simulink model "Chapter_4_Section_3_Model"  (R2017a)
settings: Solver=ode4  StartTime=0.0  StopTime=200  FixedStep=stp_sz  MaxStep=.0001  MinStep=.00005  RelTol=1e-7  AbsTol=1e-7  EnableMultiTasking=on
InitFcn:
  | load Chapter_4_Section_3
  | warning off
StopFcn:
  | save data.mat u_simulation v_simulation psi_simulation r_simulation npr_user_provided npr_achievable alpha_user_provided alpha_achievable stp_sz
  | clear all
  | load('data.mat')
  | delete('data.mat')
values from neighbouring files (symbols this model uses):
  A_disk = 13.2025431267    [Chapter_4_Section_3.mat]
  a_r11 = [-0.000865667853776 -0.901318756108 0.00874486630837 -0.00765974060328 0.00955717632387 0.00641813989061 -0.011076069832 0.00201248118094 -0.00501952733262 0.00315605586996 -0.00210851076531 0.0148609220099 ... (324 elements, 18x18)]    [Chapter_4_Section_3.mat]
  a_r13 = [-0.0294995912119 -4.91037219533 -0.00332739568397 0.0888755061346 -0.00681796875441 0.183812407485 0.0112008036726 0.10429312155 -0.0251601482875 -0.228675692165 0.00453476042855 0.0594697753606 ... (169 elements, 13x13)]    [Chapter_4_Section_3.mat]
  a_r15 = [-0.00127786555898 0.776225741104 -0.00474776997752 -0.00131066749835 0.0137520402687 -0.00211384579247 8.8019955143e-05 -0.00028996241197 -0.00129826872567 -0.0202543144732 0.0030370404199 -0.00453425604591 ... (169 elements, 13x13)]    [Chapter_4_Section_3.mat]
  a_r22 = [-0.000797108949019 -1.01015556887 0.00406573750109 -0.00111578544774 0.00423859757219 -0.00799128279013 0.00569024815652 -0.0167562674532 0.00334935655618 -0.000712432292804 0.00154242142086 0.00240437743229 ... (169 elements, 13x13)]    [Chapter_4_Section_3.mat]
  a_r24 = [-0.000686927823555 -0.95665602689 0.00244839898375 0.00145613314595 -0.00607023426216 0.0163996841317 0.00152022458075 -0.000736874734971 -0.00294919321651 -0.000761800577268 -0.00251686123035 -0.00197732815976 ... (169 elements, 13x13)]    [Chapter_4_Section_3.mat]
  a_r26 = [-0.194397873228 1.89810259721 -0.0873186628061 -0.241231729519 0.281206161775 -0.16994038615 -0.116565511469 -0.0496572593209 0.0216084469732 0.0912933167406 0.0299797727001 0.0314987707028 ... (169 elements, 13x13)]    [Chapter_4_Section_3.mat]
  a_r31 = [-0.00489112559449 -3.89960530455 -0.0361162658575 0.0265931197764 0.0034376033088 0.000316401308368 -0.0243996243526 0.0792200139858 -0.023187698537 -0.0726743997029 0.00400632061963 -0.0350516560041 ... (169 elements, 13x13)]    [Chapter_4_Section_3.mat]
  a_r33 = [-0.601431448276 0.50360246711 0.500115950342 -0.0452293844892 -0.0181314142185 -0.0323524621531 0.0355826051968 0.0329239610677 0.0940919952313 0.0566642992805 -0.0379178935102 0.0254835488846 ... (169 elements, 13x13)]    [Chapter_4_Section_3.mat]
  a_r35 = [-0.861988746714 -0.582511154549 0.34264856173 -0.0655310417272 -0.417167685168 0.183176698588 -0.473887691644 -0.225677727522 -0.133571139717 -0.218168843707 0.0850592077583 -0.0257492082836 ... (169 elements, 13x13)]    [Chapter_4_Section_3.mat]
  a_r42 = [-0.000411079312172 -0.966350953459 0.00419936729713 0.00358740198521 -0.00356571428733 -0.00958951498266 -0.00230062261745 -3.48708248632e-05 -0.00350313209064 -0.00772126326768 -0.0011918234528 -0.00149424537901 ... (169 elements, 13x13)]    [Chapter_4_Section_3.mat]
  a_r44 = [-0.000156115728087 -0.944139704333 -0.00242185567679 0.00620214191605 0.00232565005277 -0.00625050722164 0.00126021167241 -0.000681873506535 0.0011931592381 -0.00289361611357 -0.00138182415247 -0.00252837386868 ... (169 elements, 13x13)]    [Chapter_4_Section_3.mat]
  a_r46 = [-0.000218462457517 1.89677852742 0.00896242354968 -0.00290259500747 0.00225128874867 0.00254539590487 0.00120681433209 0.00261900930035 0.00149629742842 0.000796832004109 0.00199591847947 0.00352664402036 ... (169 elements, 13x13)]    [Chapter_4_Section_3.mat]
  a_r51 = [-0.0010898880101 0.776080724329 0.000225388678941 0.00375234840616 -0.00838297691459 -0.00447310416982 -0.0119510882322 -0.00692765468718 0.00227273345413 -0.0063592610709 0.000914007544175 0.00943534814934 ... (169 elements, 13x13)]    [Chapter_4_Section_3.mat]
  a_r53 = [-0.83377539904 0.569677058563 0.434285019976 0.157205409215 -0.397195569542 -0.255164078245 -0.141246880777 0.177451291189 -0.182828550566 0.0648162508754 0.244251292681 0.160100487197 ... (169 elements, 13x13)]    [Chapter_4_Section_3.mat]
  a_r55 = [-0.000352406331634 0.764343029796 0.00339830320259 -0.000678251137483 -0.00243783779313 -0.00215979913278 0.00196909451093 -0.00577428819561 -0.00349811892924 -0.00488920883323 0.00112064970343 0.000774855197444 ... (169 elements, 13x13)]    [Chapter_4_Section_3.mat]
  a_r62 = [-0.546519039316 -1.22303009993 0.393735845548 -0.120016588191 0.38151861373 -0.213578592342 -0.602267954372 -0.105716444149 -0.153151371839 -0.163939447448 -0.555540353196 0.0685401630267 ... (169 elements, 13x13)]    [Chapter_4_Section_3.mat]
  a_r64 = [-0.0406191100017 -5.18251105957 -0.115497941507 -0.0935821370219 0.180972853448 -0.0201998949456 -0.0698170640352 -0.0736823539521 -0.034828919888 0.0876659960431 -0.0419335596239 -0.0240984963396 ... (169 elements, 13x13)]    [Chapter_4_Section_3.mat]
  a_r66 = [-0.00276803466684 1.11530008029 0.0229779449181 0.0262185319857 0.00628472844795 0.000156167369042 -0.00250093023805 -0.0114435042874 -0.00826774415326 -0.00991601759993 -0.00812142854996 0.0148245002111 ... (169 elements, 13x13)]    [Chapter_4_Section_3.mat]
  A_rudder = 6    [Chapter_4_Section_3.mat]
  alpha_max = 0.392699081699    [Chapter_4_Section_3.mat]
  b_r11 = [-1.91804272115 -67.7547902158 12.3212653748 -6.25011871643 13.082442224 5.48501776184 -10.1596546398 2.56004852009 -4.74360113798 3.95981895348 -2.02856412397 18.3264246889 ... (18 elements, 18x1)]    [Chapter_4_Section_3.mat]
  b_r13 = [9.68113335046 8.54720242819 0.883931047444 -5.56576078332 1.72641800243 -13.8756826027 -2.702777864 -9.4621991361 5.92943514782 22.6516835054 -1.0074598861 -6.31102592982 ... (13 elements, 13x1)]    [Chapter_4_Section_3.mat]
  b_r22 = [-8.230214728 -263.156134326 24.2327808151 -4.87921448873 19.1715641288 -45.8768653263 26.6325387064 -91.9399975548 16.6663243552 -3.80929112747 7.68030110892 12.8381492859 ... (13 elements, 13x1)]    [Chapter_4_Section_3.mat]
  b_r24 = [20.6689502907 674.321335078 -41.3637763247 -19.2444203625 82.0775505272 -259.897803047 -22.2545830602 11.3827604156 43.2189922355 11.7516897475 36.9394390446 30.4503929007 ... (13 elements, 13x1)]    [Chapter_4_Section_3.mat]
  b_r26 = [206.794755218 -62.242559329 24.5666904254 184.158146246 -103.419961827 115.160111337 76.4499795128 20.3457431208 -13.1704465249 -41.5730935141 -18.1334448714 -14.4641153742 ... (13 elements, 13x1)]    [Chapter_4_Section_3.mat]
  b_r31 = [3.76230189948 5.16928151238 2.64945725635 -18.4251953385 -2.0625905672 -0.18887543415 4.20433084471 -14.07893046 13.0563354882 16.4007691754 -2.13849071942 8.28528512456 ... (13 elements, 13x1)]    [Chapter_4_Section_3.mat]
  b_r33 = [-425.265727934 16.4952177922 163.76327445 -15.539902078 -6.59006558263 -11.1862310226 12.8543123126 11.4260264426 33.8206936715 19.7626944669 -13.5783728882 8.91023495161 ... (13 elements, 13x1)]    [Chapter_4_Section_3.mat]
  b_r35 = [955.467057384 23.8174564739 -126.402446683 48.3788727465 168.435579445 -128.161344325 216.24493699 142.979450788 65.1193355403 134.911935543 -50.7648858119 13.1799100865 ... (13 elements, 13x1)]    [Chapter_4_Section_3.mat]
  b_r42 = [15.9360311823 665.959154186 -98.5777560157 -55.5400651809 61.9220987195 200.312325561 47.5124103398 0.631683490985 64.1219861023 155.750535985 22.3985447876 29.803792586 ... (13 elements, 13x1)]    [Chapter_4_Section_3.mat]
  b_r44 = [-27.1891200017 -1761.50772747 -283.391471232 367.311489951 182.522124626 -579.755911925 104.353356772 -62.2376848714 99.3185259533 -260.784153955 -116.536414334 -226.454300618 ... (13 elements, 13x1)]    [Chapter_4_Section_3.mat]
  b_r46 = [-26.6906838426 431.487773123 657.709356633 -144.976364483 114.646575538 180.775978583 85.0953284375 135.592940904 78.9082960716 55.2973047721 106.740201988 241.432567993 ... (13 elements, 13x1)]    [Chapter_4_Section_3.mat]
  b_r51 = [-27.9768378982 741.05041888 2.33758926296 57.3995096963 -127.005620965 -47.2947833409 -133.876425682 -98.5907202753 26.0445243962 -88.3721242204 10.7680008324 130.122749963 ... (13 elements, 13x1)]    [Chapter_4_Section_3.mat]
  b_r53 = [949.455593416 -23.2452293814 -157.318364745 -121.412853107 173.067821874 177.10214052 64.7164189373 -120.452255472 86.0623964314 -43.0643550932 -116.39314584 -105.497696438 ... (13 elements, 13x1)]    [Chapter_4_Section_3.mat]
  b_r55 = [-217.127382907 9506.32343029 1148.82922273 -188.742556573 -694.43970838 -709.996440288 566.872400877 -1877.38940059 -1026.37679575 -1566.80129668 332.089563592 247.692614281 ... (13 elements, 13x1)]    [Chapter_4_Section_3.mat]
  b_r62 = [259.61149635 16.5485296799 -38.0095496792 45.1883806678 -40.3107166739 78.3455844965 73.5107367495 37.0054960802 51.6709447748 22.7410486275 84.4875008959 -21.9559289205 ... (13 elements, 13x1)]    [Chapter_4_Section_3.mat]
  b_r64 = [156.539833252 187.686482031 376.820920142 59.4312894666 -548.902692032 17.0176436095 70.7484878223 206.821047291 37.1716677759 -243.032149857 114.824775027 27.0037475025 ... (13 elements, 13x1)]    [Chapter_4_Section_3.mat]
  b_r66 = [-314.266256408 5285.46587095 1093.01941502 1627.30071258 387.633965073 8.0986510694 -130.443621448 -701.343286032 -436.49966457 -600.0481003 -433.735518303 884.367320612 ... (13 elements, 13x1)]    [Chapter_4_Section_3.mat]
  bettas_CQ = [0 5.39 17.77 34.97 50.79 58.7 64.55 68.33 73.49 85.2 93.11 102.75 ... (40 elements, 1x40)]    [Chapter_4_Section_3.mat]    (also in looking_up_n.m = [0 5.39 17.77 34.97 50.79 58.7 64.55 68.33 73.49 85.2 93.11 )
  bettas_CT = [0 5.37 16.73 33.6 44.63 60.82 73.22 80.46 86.3 92.15 100.41 110.74 ... (52 elements, 1x52)]    [Chapter_4_Section_3.mat]    (also in looking_up_n.m = [0 5.37 16.73 33.6 44.63 60.82 73.22 80.46 86.3 92.15 100.41)
  c_r11 = [1.91804272142 -67.7547902158 -12.3212653748 -6.25011871643 -13.082442224 5.48501776185 -10.1596546398 -2.56004852009 -4.74360113798 -3.95981895348 -2.02856412396 -18.3264246889 ... (18 elements, 1x18)]    [Chapter_4_Section_3.mat]
  c_r13 = [9.68113335045 -8.54720242824 0.883931047418 5.56576078332 1.72641800244 13.8756826027 -2.702777864 9.4621991361 5.92943514781 -22.6516835054 -1.0074598861 6.31102592982 ... (13 elements, 1x13)]    [Chapter_4_Section_3.mat]
  c_r22 = [8.23021472807 -263.156134326 -24.2327808151 -4.87921448871 19.1715641288 45.8768653263 26.6325387064 91.9399975548 16.6663243552 3.80929112749 7.68030110892 -12.8381492859 ... (13 elements, 1x13)]    [Chapter_4_Section_3.mat]
  c_r24 = [20.6689502903 -674.321335078 -41.3637763247 19.2444203625 -82.0775505271 -259.897803047 22.2545830602 11.3827604156 -43.2189922355 11.7516897475 -36.9394390446 30.4503929007 ... (13 elements, 1x13)]    [Chapter_4_Section_3.mat]
  c_r26 = [-206.794755218 -62.2425593289 24.5666904254 -184.158146246 -103.419961827 -115.160111337 -76.4499795128 20.3457431209 13.1704465249 -41.5730935141 18.1334448714 -14.4641153742 ... (13 elements, 1x13)]    [Chapter_4_Section_3.mat]
  c_r31 = [3.76230189951 -5.16928151238 -2.64945725636 -18.4251953385 -2.0625905672 -0.188875434257 -4.2043308447 14.07893046 13.0563354882 -16.4007691754 -2.13849071943 -8.28528512456 ... (13 elements, 1x13)]    [Chapter_4_Section_3.mat]
  c_r33 = [-425.265727934 -16.4952177923 -163.76327445 15.539902078 -6.5900655826 11.1862310226 12.8543123126 -11.4260264426 33.8206936715 -19.7626944669 -13.5783728882 -8.91023495161 ... (13 elements, 1x13)]    [Chapter_4_Section_3.mat]
  c_r35 = [-955.467057384 23.8174564746 -126.402446683 -48.3788727464 168.435579445 128.161344325 216.24493699 -142.979450788 65.1193355403 -134.911935543 50.7648858119 13.1799100865 ... (13 elements, 1x13)]    [Chapter_4_Section_3.mat]
  c_r42 = [15.9360311824 -665.959154186 -98.5777560157 55.5400651809 -61.9220987195 200.312325561 47.5124103398 -0.631683490192 -64.1219861023 155.750535985 -22.3985447876 29.803792586 ... (13 elements, 1x13)]    [Chapter_4_Section_3.mat]
  c_r44 = [27.189120009 -1761.50772747 283.391471232 367.311489951 182.522124626 579.755911925 104.353356772 62.2376848713 99.3185259533 260.784153955 -116.536414334 226.454300618 ... (13 elements, 1x13)]    [Chapter_4_Section_3.mat]
  c_r46 = [26.6906838375 431.487773123 -657.709356633 -144.976364484 114.646575538 -180.775978583 -85.0953284373 135.592940904 78.9082960717 -55.297304772 106.740201988 -241.432567993 ... (13 elements, 1x13)]    [Chapter_4_Section_3.mat]
  c_r51 = [27.9768378982 741.05041888 2.33758926325 -57.3995096963 127.005620965 -47.2947833409 -133.876425682 98.5907202753 26.0445243962 88.3721242204 10.7680008324 -130.122749963 ... (13 elements, 1x13)]    [Chapter_4_Section_3.mat]
  c_r53 = [-949.455593416 -23.2452293814 -157.318364745 121.412853107 173.067821874 -177.10214052 64.7164189374 120.452255472 86.0623964314 43.0643550932 -116.39314584 105.497696438 ... (13 elements, 1x13)]    [Chapter_4_Section_3.mat]
  c_r55 = [217.12738291 9506.32343029 -1148.82922273 -188.742556576 -694.43970838 709.996440288 566.872400876 1877.38940059 -1026.37679575 1566.80129668 332.089563594 -247.69261428 ... (13 elements, 1x13)]    [Chapter_4_Section_3.mat]
  c_r62 = [-259.61149635 16.5485296799 -38.0095496792 -45.1883806678 -40.3107166739 -78.3455844965 73.5107367495 -37.0054960802 -51.6709447748 22.7410486275 84.4875008959 21.9559289205 ... (13 elements, 1x13)]    [Chapter_4_Section_3.mat]
  c_r64 = [-156.539833251 187.686482031 -376.820920142 59.4312894666 548.902692032 17.0176436097 70.7484878223 -206.82104729 37.1716677758 243.032149857 -114.824775027 27.0037475025 ... (13 elements, 1x13)]    [Chapter_4_Section_3.mat]
  c_r66 = [314.266256408 5285.46587095 1093.01941502 -1627.30071258 -387.633965073 8.09865107118 -130.443621448 701.343286032 -436.49966457 600.0481003 -433.735518303 -884.367320612 ... (13 elements, 1x13)]    [Chapter_4_Section_3.mat]
  CQs = [0.008 0.007 -0.002 -0.018 -0.037 -0.049 -0.06 -0.065 -0.068 -0.059 -0.057 -0.059 ... (40 elements, 1x40)]    [Chapter_4_Section_3.mat]    (also in looking_up_n.m = -0.1.*[-0.08 -0.07 0.02 0.18 0.37 0.49 0.6 0.65 0.68 0.59 0.)
  CTs = [0.32 0.29 0.19 0.01 -0.16 -0.46 -0.7 -0.77 -0.7 -0.63 -0.63 -0.69 ... (52 elements, 1x52)]    [Chapter_4_Section_3.mat]    (also in looking_up_n.m = [0.32 0.29 0.19 0.01 -0.16 -0.46 -0.7 -0.77 -0.7 -0.63 -0.63)
  d_r11 = 95.5285227708    [Chapter_4_Section_3.mat]
  d_r13 = -14.1628545989    [Chapter_4_Section_3.mat]
  d_r22 = 1468.51041279    [Chapter_4_Section_3.mat]
  d_r24 = -9785.77027698    [Chapter_4_Section_3.mat]
  d_r26 = -1700.92421833    [Chapter_4_Section_3.mat]
  d_r31 = -0.95522945761    [Chapter_4_Section_3.mat]
  d_r33 = 3827.81220596    [Chapter_4_Section_3.mat]
  d_r35 = -19539.5268707    [Chapter_4_Section_3.mat]
  d_r42 = -9418.04264727    [Chapter_4_Section_3.mat]
  d_r44 = 68252.1479072    [Chapter_4_Section_3.mat]
  d_r46 = -10162.1377852    [Chapter_4_Section_3.mat]
  d_r51 = 12054.4514237    [Chapter_4_Section_3.mat]
  d_r53 = -19539.5038011    [Chapter_4_Section_3.mat]
  d_r55 = 1991036.95813    [Chapter_4_Section_3.mat]
  d_r62 = -1405.47636444    [Chapter_4_Section_3.mat]
  d_r64 = -12342.2523681    [Chapter_4_Section_3.mat]
  d_r66 = 610786.440495    [Chapter_4_Section_3.mat]
  DEN = 5.34671106464e+28    [Chapter_4_Section_3.mat]
  dist_LOS = [-50 -49 -48 -47 -46 -45 -44 -43 -42 -41 -40 -39 ... (1051 elements, 1x1051)]    [Chapter_4_Section_3.mat]
  Dpr = 4.1    [Chapter_4_Section_3.mat]    (also in looking_up_n.m = u(4))
  Dw = 0.110526315789    [Chapter_4_Section_3.mat]
  dx = 10    [Chapter_4_Section_3.mat]
  dxr = 48.75    [Chapter_4_Section_3.mat]
  dy = 2    [Chapter_4_Section_3.mat]
  dz = 0.8    [Chapter_4_Section_3.mat]
  dzr = 0.514285714286    [Chapter_4_Section_3.mat]
  g = 10    [Chapter_4_Section_3.mat]
  gravity = 10    [Chapter_4_Section_3.mat]
  INDEX = [1 2 3 4 5 6 7 8 9]    [Chapter_4_Section_3.mat]
  Ix = 724554000    [Chapter_4_Section_3.mat]
  Iy = 4528460000    [Chapter_4_Section_3.mat]
  Iz = 4528460000    [Chapter_4_Section_3.mat]
  k_wave = [0.0157865285852 0.0224311321394 0.0345394916241 0.0578593033576 0.0778685019714 0.0983501894009 0.10403521245 0.134043066308 0.155236404606 0.203205074918 0.220032771713 0.262178651673 ... (20 elements, 1x20)]    [Chapter_4_Section_3.mat]
  Last_Pt_Accuracy = 30    [Chapter_4_Section_3.mat]
  LBP = 100    [Chapter_4_Section_3.mat]
  m = 7264000    [Chapter_4_Section_3.mat]
  phase = [4.61787442739 6.09845039199 5.44708367148 0.54182753101 2.30238916367 2.31974450279 4.30416083443 3.75697809799 4.95971993271 2.31003141527 1.29451121971 0.54454197722 ... (20 elements, 1x20)]    [Chapter_4_Section_3.mat]
  phi_0 = 0    [Chapter_4_Section_3.mat]
  psi_0 = 0    [Chapter_4_Section_3.mat]
  R_convrg = 220    [Chapter_4_Section_3.mat]
  radius_LOS = [166.575605377 166.637026665 166.698699321 166.760625342 166.82280675 166.885245588 166.947943925 167.010903854 167.074127493 167.137616985 167.201374499 167.265402228 ... (1051 elements, 1x1051)]    [Chapter_4_Section_3.mat]
  raw = 1000    [Chapter_4_Section_3.mat]    (also in looking_up_n.m = u(3))
  s = 0.15    [Chapter_4_Section_3.mat]
  S11 = 5.22457985714e+28    [Chapter_4_Section_3.mat]
  S13 = 3.79917831589e+26    [Chapter_4_Section_3.mat]
  S15 = -4.97006200608e+19    [Chapter_4_Section_3.mat]
  S22 = 4.58630932583e+28    [Chapter_4_Section_3.mat]
  S24 = 9.38800137353e+19    [Chapter_4_Section_3.mat]
  S26 = 1.30387886946e+18    [Chapter_4_Section_3.mat]
  S31 = 3.83422033136e+26    [Chapter_4_Section_3.mat]
  S33 = 1.77296018417e+28    [Chapter_4_Section_3.mat]
  S35 = 2.44593333777e+19    [Chapter_4_Section_3.mat]
  S42 = 8.93369784557e+19    [Chapter_4_Section_3.mat]
  S44 = 7.37931315974e+19    [Chapter_4_Section_3.mat]
  S46 = 27990784014.6    [Chapter_4_Section_3.mat]
  S51 = -4.98658939538e+19    [Chapter_4_Section_3.mat]
  S53 = 2.45188465874e+19    [Chapter_4_Section_3.mat]
  S55 = 1.18069051188e+19    [Chapter_4_Section_3.mat]
  S62 = 1.30580221388e+18    [Chapter_4_Section_3.mat]
  S64 = 23535167243.9    [Chapter_4_Section_3.mat]
  S66 = 1.18069078235e+19    [Chapter_4_Section_3.mat]
  ... (+18 more)
undefined symbols (not defined in the file or in its folder): magnitude
libraries: simulink x9
(part 6 of 6)

== system Chapter_4_Section_3_Model/Ship_Model/Ship Dynamics with Environmental Forces and Memory Effect/Buoyancy_Forces/Subsystem/wave elevation from multiple frequencies/Seakeeping motion of the ship from RAO's and wave spectrum /Sea wave elevation from  ==
  w_star : Inport
  k_wave : Inport  Port=2
  phase : Inport  Port=3
  X : Inport  Port=4
  Y : Inport  Port=5
  t : Inport  Port=6
  S_power of ith wave : Inport  Port=7
  ksi : Inport  Port=8
  Math Function : Math  Operator=sqrt  SaturateOnIntegerOverflow=on
  Product{,2..5} (5 alike) : Product  RndMeth=Zero
  Product1 : Product  Inputs=3  RndMeth=Zero
  Read Me : simulink/Model-Wide Utilities/DocBlock  DocumentType=Text
  Sum : Sum  Inputs=|+|+|-|
  Sum1 : Sum  Inputs=|+|+|
  Trigonometric Function : Trigonometry  Operator=cos
  Trigonometric Function1 : Trigonometry
  Trigonometric Function2 : Trigonometry  Operator=cos
  transforming Y to the z-upward -inertial frame(our inertial frame has z-downwards) : Gain  Gain=-1
  transforming the wave elevation from wave frame to  our inertial frame that has z-downwards : Gain  Gain=-1
  w12 : Constant  Value=2
  w13 : Constant  Value=Dw
  Sea wave Elevation(m) : Outport
  wires:
  transforming the wave elevation from wave frame to  our inertial frame that has z-downwards/1 -> Sea wave Elevation(m)/1
  transforming Y to the z-upward -inertial frame(our inertial frame has z-downwards)/1 -> [Y]
  Product5/1 -> transforming the wave elevation from wave frame to  our inertial frame that has z-downwards/1
  Trigonometric Function2/1 -> Product5/2
  Math Function/1 -> Product5/1
  Product1/1 -> Math Function/1
  [Dw] -> Product1/3
  [S] -> Product1/2
  w12/1 -> Product1/1
  Sum/1 -> Trigonometric Function2/1
  w13/1 -> [Dw]
  Product4/1 -> Sum/3
  [k_wave] -> Product4/1
  Sum1/1 -> Product4/2
  Product3/1 -> Sum1/2
  Product2/1 -> Sum1/1
  Trigonometric Function1/1 -> Product3/2
  [Y] -> Product3/1
  Trigonometric Function/1 -> Product2/2
  [X] -> Product2/1
  ksi/1 -> Trigonometric Function/1, Trigonometric Function1/1
  Y/1 -> transforming Y to the z-upward -inertial frame(our inertial frame has z-downwards)/1
  X/1 -> [X]
  phase/1 -> [phase]
  k_wave/1 -> [k_wave]
  w_star/1 -> [w_star]
  [phase] -> Sum/2
  Product/1 -> Sum/1
  [t] -> Product/2
  [w_star] -> Product/1
  t/1 -> [t]
  S_power of ith wave/1 -> [S]

== system Chapter_4_Section_3_Model/Ship_Model/Ship Dynamics with Environmental Forces and Memory Effect/Buoyancy_Forces/Subsystem/wave elevation from multiple frequencies1/Seakeeping motion of the ship from RAO's and wave spectrum /Sea wave elevation from  ==
  w_star : Inport
  k_wave : Inport  Port=2
  phase : Inport  Port=3
  X : Inport  Port=4
  Y : Inport  Port=5
  t : Inport  Port=6
  S_power of ith wave : Inport  Port=7
  ksi : Inport  Port=8
  Math Function : Math  Operator=sqrt  SaturateOnIntegerOverflow=on
  Product{,2..5} (5 alike) : Product  RndMeth=Zero
  Product1 : Product  Inputs=3  RndMeth=Zero
  Read Me : simulink/Model-Wide Utilities/DocBlock  DocumentType=Text
  Sum : Sum  Inputs=|+|+|-|
  Sum1 : Sum  Inputs=|+|+|
  Trigonometric Function : Trigonometry  Operator=cos
  Trigonometric Function1 : Trigonometry
  Trigonometric Function2 : Trigonometry  Operator=cos
  transforming Y to the z-upward -inertial frame(our inertial frame has z-downwards) : Gain  Gain=-1
  transforming the wave elevation from wave frame to  our inertial frame that has z-downwards : Gain  Gain=-1
  w12 : Constant  Value=2
  w13 : Constant  Value=Dw
  Sea wave Elevation(m) : Outport
  wires:
  transforming the wave elevation from wave frame to  our inertial frame that has z-downwards/1 -> Sea wave Elevation(m)/1
  transforming Y to the z-upward -inertial frame(our inertial frame has z-downwards)/1 -> [Y]
  Product5/1 -> transforming the wave elevation from wave frame to  our inertial frame that has z-downwards/1
  Trigonometric Function2/1 -> Product5/2
  Math Function/1 -> Product5/1
  Product1/1 -> Math Function/1
  [Dw] -> Product1/3
  [S] -> Product1/2
  w12/1 -> Product1/1
  Sum/1 -> Trigonometric Function2/1
  w13/1 -> [Dw]
  Product4/1 -> Sum/3
  [k_wave] -> Product4/1
  Sum1/1 -> Product4/2
  Product3/1 -> Sum1/2
  Product2/1 -> Sum1/1
  Trigonometric Function1/1 -> Product3/2
  [Y] -> Product3/1
  Trigonometric Function/1 -> Product2/2
  [X] -> Product2/1
  ksi/1 -> Trigonometric Function/1, Trigonometric Function1/1
  Y/1 -> transforming Y to the z-upward -inertial frame(our inertial frame has z-downwards)/1
  X/1 -> [X]
  phase/1 -> [phase]
  k_wave/1 -> [k_wave]
  w_star/1 -> [w_star]
  [phase] -> Sum/2
  Product/1 -> Sum/1
  [t] -> Product/2
  [w_star] -> Product/1
  t/1 -> [t]
  S_power of ith wave/1 -> [S]

== matlab function Chapter_4_Section_3_Model/Ship_Model/Ship Dynamics with Environmental Forces and Memory Effect/Six DOF State Integrator of the Ship/J2 matrix ==
  data: u input; y output
function y = J2(u)
% This block supports an embeddable subset of the MATLAB language.
% See the help menu for details. 
y=[1 sin(u(1))*tan(u(2)) cos(u(1))*tan(u(2));0 cos(u(1)) -sin(u(1));0 sin(u(1))/cos(u(2)) cos(u(1))/cos(u(2))];

== matlab function Chapter_4_Section_3_Model/Ship_Model/Ship Dynamics with Environmental Forces and Memory Effect/Six DOF State Integrator of the Ship/J1 matrix ==
  data: u input; y output
function y = J1(u)
% This block supports an embeddable subset of the MATLAB language.
% See the help menu for details. 
y=[cos(u(3))*cos(u(2))    -sin(u(3))*cos(u(1))+cos(u(3))*sin(u(2))*sin(u(1))   sin(u(3))*sin(u(1))+cos(u(3))*cos(u(1))*sin(u(2))  ;    ...
    sin(u(3))*cos(u(2))           cos(u(3))*cos(u(1))+ sin(u(1))*sin(u(2))*sin(u(3))    -cos(u(3))*sin(u(1))+sin(u(2))*sin(u(3))*cos(u(1))  ; ... 
-sin(u(2))                                             cos(u(2))*sin(u(1))                                                                 cos(u(2))*cos(u(1)) ];

== matlab function Chapter_4_Section_3_Model/Ship_Model/Ship Dynamics with Environmental Forces and Memory Effect/Buoyancy_Forces/J1 matrix ==
  data: u input; y output
function y = J1(u)
% This block supports an embeddable subset of the MATLAB language.
% See the help menu for details. 
y=inv(u);

== matlab function Chapter_4_Section_3_Model/Ship_Model/Ship Dynamics with Environmental Forces and Memory Effect/Wave Excitation Force/wave elevation from multiple frequencies2/Seakeeping motion of the ship from RAO's and wave spectrum /Embedded MATLAB Function ==
  data: index input; y output; A input
function y = fcn(index,A)
% This block supports an embeddable subset of the MATLAB language.
% See the help menu for details. 
y =A(index);

== matlab function Chapter_4_Section_3_Model/Ship_Model/Ship Dynamics with Environmental Forces and Memory Effect/Wave Excitation Force/wave elevation from multiple frequencies2/Seakeeping motion of the ship from RAO's and wave spectrum /Embedded MATLAB Function1 ==
  data: index input; y output; A input
function y = fcn(index,A)
% This block supports an embeddable subset of the MATLAB language.
% See the help menu for details. 
y =A(index);

== matlab function Chapter_4_Section_3_Model/Ship_Model/Ship Dynamics with Environmental Forces and Memory Effect/Buoyancy_Forces/Subsystem/wave elevation from multiple frequencies1/Seakeeping motion of the ship from RAO's and wave spectrum /Embedded MATLAB Function ==
  data: index input; y output; A input
function y = fcn(index,A)
% This block supports an embeddable subset of the MATLAB language.
% See the help menu for details. 
y =A(index);

== matlab function Chapter_4_Section_3_Model/Ship_Model/Ship Dynamics with Environmental Forces and Memory Effect/Buoyancy_Forces/Subsystem/wave elevation from multiple frequencies1/Seakeeping motion of the ship from RAO's and wave spectrum /Embedded MATLAB Function1 ==
  data: index input; y output; A input
function y = fcn(index,A)
% This block supports an embeddable subset of the MATLAB language.
% See the help menu for details. 
y =A(index);

== matlab function Chapter_4_Section_3_Model/Ship_Model/Ship Dynamics with Environmental Forces and Memory Effect/Buoyancy_Forces/Subsystem/J1 matrix ==
  data: u input; y output
function y = J1(u)
% This block supports an embeddable subset of the MATLAB language.
% See the help menu for details. 
y=u(1,:)   ;

== matlab function Chapter_4_Section_3_Model/Ship_Model/Ship Dynamics with Environmental Forces and Memory Effect/Buoyancy_Forces/Subsystem/J1 matrix1 ==
  data: u input; y output
function y = J1(u)
% This block supports an embeddable subset of the MATLAB language.
% See the help menu for details. 
y=u(2,:)   ;

== matlab function Chapter_4_Section_3_Model/Ship_Model/Ship Dynamics with Environmental Forces and Memory Effect/Buoyancy_Forces/Subsystem/wave elevation from multiple frequencies1/Seakeeping motion of the ship from RAO's and wave spectrum /Embedded MATLAB Function2 ==
  data: index input; y output; A input
function y = fcn(index,A)
% This block supports an embeddable subset of the MATLAB language.
% See the help menu for details. 
y =A(index);

== matlab function Chapter_4_Section_3_Model/Ship_Model/Ship Dynamics with Environmental Forces and Memory Effect/Wave Excitation Force/wave elevation from multiple frequencies2/Seakeeping motion of the ship from RAO's and wave spectrum /Embedded MATLAB Function2 ==
  data: index input; y output; A input
function y = fcn(index,A)
% This block supports an embeddable subset of the MATLAB language.
% See the help menu for details. 
y =A(index);

== matlab function Chapter_4_Section_3_Model/Ship_Model/LOS2/Breivik Model for psi/pi2inf ==
  data: x_los input; state_k output; y_los input; x input; y input; state_k_1 input; psi_k_1 input; psi_k input; accumulation_k_1 input; accumulation_k output
function [state_k ,accumulation_k]= fcn(x_los,y_los,x,y,state_k_1,psi_k_1,psi_k,accumulation_k_1)
delta_x = x_los - x;
delta_y = y_los- y;


% initialize:
accumulation_k = accumulation_k_1;
state_k=state_k_1;
% if( sign(delta_y)==1 && sign(delta_x)==1 )
if( sign(delta_y)>=0 && sign(delta_x)>=0 )
    % Now in the 1.quadrant
    state_k=1;
    if(state_k_1==3)
        if( (psi_k+abs(psi_k_1))<=pi )
            accumulate = psi_k - psi_k_1;
        else
            accumulate = psi_k_1 - psi_k + 2*pi;
        end
    else % state_k_1 == 1, 2 or 4
        accumulate = psi_k - psi_k_1;
    end
% elseif ( sign(delta_y)==-1 && sign(delta_x)==1 )
elseif ( sign(delta_y)<=0 && sign(delta_x)>=0 )
    % Now in the 2.quadrant
    state_k=2;
    if(state_k_1==4)
        if( (abs(psi_k)+psi_k_1)<=pi )
            accumulate = psi_k - psi_k_1;
        else
            accumulate = psi_k - psi_k_1 + 2*pi;
        end
    else % state_k_1 == 1, 2 or 3
        accumulate = psi_k - psi_k_1;
    end
% elseif (sign(delta_y)==-1 && sign(delta_x)==-1 )
elseif (sign(delta_y)<0 && sign(delta_x)<=0 )
    % Now in the 3.quadrant
    state_k=3;
    if(state_k_1==1)
        if( (abs(psi_k)+psi_k_1)<=pi )
            accumulate = psi_k - psi_k_1;
        else
            accumulate = psi_k - psi_k_1 + 2*pi;
        end
    elseif(state_k_1==4)
        accumulate = psi_k - psi_k_1 + 2*pi;
    else % state_k_1 == 2 or 3
        accumulate = psi_k - psi_k_1;
    end
else
    % sign(delta_y)==1 && sign(delta_x)==-1
    % Now in the 4.quadrant
    state_k=4;
    if(state_k_1==2)
        if( (psi_k+abs(psi_k_1))<=pi )
            accumulate = psi_k - psi_k_1;
        else
            accumulate = psi_k_1 - psi_k + 2*pi;
        end
    elseif(state_k_1==3)
        accumulate = psi_k - psi_k_1 - 2*pi;
    else % state_k_1 == 1 or 4
        accumulate = psi_k - psi_k_1;
    end
end
accumulation_k = accumulation_k_1 + accumulate;

if isreal(accumulation_k)==0
    accumulation_k =accumulation_k_1
end

if isreal(state_k )==0
    state_k =state_k_1
end
if length(state_k)>1
    state_k=state_k(1);
end
if length(accumulation_k)>1
    accumulation_k=accumulation_k(1);
end

if isnan(accumulation_k)==1
    accumulation_k =accumulation_k_1;
end

if isnan(state_k )==1
    state_k =state_k_1;
end

% Y = [state_k ;accumulation_k];

== matlab function Chapter_4_Section_3_Model/Ship_Model/Ship Dynamics with Environmental Forces and Memory Effect/Buoyancy_Forces/Subsystem/wave elevation from multiple frequencies1/Seakeeping motion of the ship from RAO's and wave spectrum /Embedded MATLAB Function3 ==
  data: index input; y output; A input
function y = fcn(index,A)
% This block supports an embeddable subset of the MATLAB language.
% See the help menu for details. 
y =A(index);

== matlab function Chapter_4_Section_3_Model/Ship_Model/Ship Dynamics with Environmental Forces and Memory Effect/Buoyancy_Forces/Subsystem/wave elevation from multiple frequencies/Seakeeping motion of the ship from RAO's and wave spectrum /Embedded MATLAB Function3 ==
  data: index input; y output; A input
function y = fcn(index,A)
% This block supports an embeddable subset of the MATLAB language.
% See the help menu for details. 
y =A(index);

== matlab function Chapter_4_Section_3_Model/Ship_Model/Ship Dynamics with Environmental Forces and Memory Effect/Wave Excitation Force/wave elevation from multiple frequencies2/Seakeeping motion of the ship from RAO's and wave spectrum /Embedded MATLAB Function3 ==
  data: index input; y output; A input
function y = fcn(index,A)
% This block supports an embeddable subset of the MATLAB language.
% See the help menu for details. 
y =A(index);

== matlab function Chapter_4_Section_3_Model/Ship_Model/Ship Dynamics with Environmental Forces and Memory Effect/Buoyancy_Forces/Subsystem/J1 matrix2 ==
  data: u input; y output
function y = J1(u)
% This block supports an embeddable subset of the MATLAB language.
% See the help menu for details. 
y=u(3,:)   ;

== matlab function Chapter_4_Section_3_Model/Ship_Model/LOS2/Subsystem1/Computing the intersection between the line and the circle1 ==
  data: x input; y input; x_i input; y_i input; x_i1 input; y_i1 input; x_los output; R input; y_los output
function [x_los,y_los]=LOS_new(x,y,x_i,y_i,x_i1,y_i1,R)
% flag=1000=> no intersection
%flag=2000=>interesction outside the segment [AB]

k=(y_i1-y_i)/(x_i1-x_i);
flag=1;
x_los=0;
y_los=0;
if x_i1==x_i
    x_los=x_i;
    if abs(x-x_i)<R
        if y_i1>y_i
            y_los=y+sqrt(R^2-(x_i-x)^2);
            flag=1;
        else
            y_los=y-sqrt(R^2-(x_i-x)^2);
            flag=2;
        end
    elseif abs(x-x_i)==R
        flag=3;
        y_los=y;
    else %abs(x-x_i)<R =>no intersection
        y_los=inf;
        flag=1000;
    end
else
      a=(1+k^2);
      b=-2*x-2*k^2*x_i+2*k*y_i-2*k*y;
      c=(x^2+k^2*x_i^2+y_i^2-2*y_i*y+y^2-2*k*x_i*y_i+2*k*x_i*y-R^2);
      delta=b^2-4*a*c;
      if delta<0
          flag=1000;
          x_los=inf;
          y_los=inf;
      elseif delta==0
          flag=4;
          x_los=(-b)/(2*a);
          y_los=k*(x_los-x_i)+y_i;
          if (x_los-x_i)*(x_los-x_i1)>0 || (y_los-y_i)*(y_los-y_i1)>0
              flag=2000;
          end
      else 
          if (x_i1-x_i)>0
              flag=5;
              x_los=(-b+sqrt(delta))/(2*a);
          else 
              flag=6;
              x_los=(-b-sqrt(delta))/(2*a);
          end
          y_los=k*(x_los-x_i)+y_i;
          if (x_los-x_i)*(x_los-x_i1)>0 || (y_los-y_i)*(y_los-y_i1)>0
              flag=2000;
          end
      end
end
% 
if (x_i~=x_los) && (y_i~=y_los)
if (x_i1-x_los)/(x_i-x_los)>1 || (y_i1-y_los)/(y_i-y_los)>1 %this condition eliminates the presence of a point lying outside the path line Ai Ai+1
         x_los=x_i;                                                               %from the side of Ai
         y_los=y_i;
end
end
%

== matlab function Chapter_4_Section_3_Model/Ship_Model/Ship Dynamics with Environmental Forces and Memory Effect/Buoyancy_Forces/Subsystem/wave elevation from multiple frequencies/Seakeeping motion of the ship from RAO's and wave spectrum /Embedded MATLAB Function ==
  data: index input; y output; A input
function y = fcn(index,A)
% This block supports an embeddable subset of the MATLAB language.
% See the help menu for details. 
y =A(index);

== matlab function Chapter_4_Section_3_Model/Ship_Model/Ship Dynamics with Environmental Forces and Memory Effect/Buoyancy_Forces/Subsystem/wave elevation from multiple frequencies/Seakeeping motion of the ship from RAO's and wave spectrum /Embedded MATLAB Function1 ==
  data: index input; y output; A input
function y = fcn(index,A)
% This block supports an embeddable subset of the MATLAB language.
% See the help menu for details. 
y =A(index);

== matlab function Chapter_4_Section_3_Model/Ship_Model/Ship Dynamics with Environmental Forces and Memory Effect/Buoyancy_Forces/Subsystem/wave elevation from multiple frequencies/Seakeeping motion of the ship from RAO's and wave spectrum /Embedded MATLAB Function2 ==
  data: index input; y output; A input
function y = fcn(index,A)
% This block supports an embeddable subset of the MATLAB language.
% See the help menu for details. 
y =A(index);

== matlab function Chapter_4_Section_3_Model/Ship_Model/Ship Dynamics with Environmental Forces and Memory Effect/Wind Force/wind force/Embedded MATLAB Function2 ==
  data: Wind_angle input; Cxw output; Ship_type input; Cyw output; CNw output
% This function computes the three wind coefficients based on Isherwood's
% method 1973 if the parameters of the ship are unknown.
%       Wind_angle: angle of attack of the wind given in degrees
%       Ship_type: integer between [1,11] indicating the type of the ship. 
% [Cxw, Cyw, CNw]=wind_coefficients_1([30,5])
function [Cxw, Cyw, CNw]=wind_coefficients_2(Wind_angle,Ship_type)

% if ceil(Ship_type)-floor(Ship_type)~=0
%     msgbox('Ship type must be an integer between [1,11]','Error','error');
% elseif Ship_type>11 ||   Ship_type<1
%     msgbox('Ship type must be an integer between [1,11]','Error','error');
% end
% Ship Type        D1  D2  D3  D4 D5  D6  M
D=[...
    1 0.192 1.95 7.66 1.44 0.492 0.398 2;...
    2 0.111 1.67 7.80 1.51 0.490 0.258 4;...
    3 0.149 2.04 7.80 1.58 0.489 0.188 0;...
    4 0.122 1.75 7.80 1.51 0.550 0.253 0;...
    5 0.151 2.06 7.80 1.58 0.526 0.175 5;...
    6 0.076 1.03 7.46 1.33 0.547 0.252 3;...
    7 0.117 1.43 7.46 1.40 0.522 0.161 0;...
    8 0.100 1.59 7.46 1.33 0.568 0.211 0;...
    9 0.121 1.68 7.46 1.40 0.537 0.139 0;...
    10 0.166 1.80 6.47 1.45 0.476 0.229 0;...
    11 0.236 1.43 4.05 1.86 0.405 0.396 1];
D1=D(Ship_type,2);
D2=D(Ship_type,3);
D3=D(Ship_type,4);
D4=D(Ship_type,5);
D5=D(Ship_type,6);
D6=D(Ship_type,7);
M=D(Ship_type,8);


%angle(DEGREE)    A0 A1 A2 A3 A4 A5 A6 STANDARD ERROR
A=...
   [0    2.1520   -5.0000    0.2430   -0.1640         0         0         0    0.0860;...
   10.0000    1.7140   -3.3300    0.1450   -0.1210         0         0         0    0.1040;...
   20.0000    1.8180   -3.9700    0.2110   -0.1430         0         0    0.0330    0.0960;...
   30.0000    1.9650   -4.8100    0.2430   -0.1540         0         0    0.0410    0.1170;...
   40.0000    2.3330   -5.9900    0.2470   -0.1900         0         0    0.0420    0.1150;...
   50.0000    1.7260   -6.5400    0.1890   -0.1730    0.3480         0    0.0480    0.1090;...
   60.0000    0.9130   -4.6800         0   -0.1040    0.4820         0    0.0520    0.0820;...
   70.0000    0.4570   -2.8800         0   -0.0680    0.3460         0    0.0430    0.0770;...
   80.0000    0.3410   -0.9100         0   -0.0310         0         0    0.0320    0.0900;...
   90.0000    0.3550         0         0         0   -0.2470         0    0.0180    0.0940;...
  100.0000    0.6010         0         0         0   -0.3720         0   -0.0202    0.0960;...
  110.0000    0.6510    1.2900         0         0   -0.5820         0   -0.0310    0.0900;...
  120.0000    0.5640    2.5400         0         0   -0.7480         0   -0.0240    0.1000;...
  130.0000   -0.1420    3.5800         0    0.0470   -0.7000         0   -0.0280    0.1050;...
  140.0000   -0.6770    3.6400         0    0.0690   -0.5290         0   -0.0320    0.1230;...
  150.0000   -0.7230    3.1400         0    0.0640   -0.4750         0   -0.0320    0.1280;...
  160.0000   -2.1480    2.5600         0    0.0810         0    1.2700   -0.0270    0.1230;...
  170.0000   -2.7070    3.9700   -0.1750    0.1260         0    1.8100         0    0.1150;...
  180.0000   -2.5290    3.7600   -0.1740    0.1280         0    1.5500         0    0.1120;...
  190.0000   -2.7070    3.9700   -0.1750    0.1260         0    1.8100         0    0.1150;...
  200.0000   -2.1480    2.5600         0    0.0810         0    1.2700   -0.0270    0.1230;...
  210.0000   -0.7230    3.1400         0    0.0640   -0.4750         0   -0.0320    0.1280;...
  220.0000   -0.6770    3.6400         0    0.0690   -0.5290         0   -0.0320    0.1230;...
  230.0000   -0.1420    3.5800         0    0.0470   -0.7000         0   -0.0280    0.1050;...
  240.0000    0.5640    2.5400         0         0   -0.7480         0   -0.0240    0.1000;...
  250.0000    0.6510    1.2900         0         0   -0.5820         0   -0.0310    0.0900;...
  260.0000    0.6010         0         0         0   -0.3720         0   -0.0202    0.0960;...
  270.0000    0.3550         0         0         0   -0.2470         0    0.0180    0.0940;...
  280.0000    0.3410   -0.9100         0   -0.0310         0         0    0.0320    0.0900;...
  290.0000    0.4570   -2.8800         0   -0.0680    0.3460         0    0.0430    0.0770;...
  300.0000    0.9130   -4.6800         0   -0.1040    0.4820         0    0.0520    0.0820;...
  310.0000    1.7260   -6.5400    0.1890   -0.1730    0.3480         0    0.0480    0.1090;...
  320.0000    2.3330   -5.9900    0.2470   -0.1900         0         0    0.0420    0.1150;...
  330.0000    1.9650   -4.8100    0.2430   -0.1540         0         0    0.0410    0.1170;...
  340.0000    1.8180   -3.9700    0.2110   -0.1430         0         0    0.0330    0.0960;...
  350.0000    1.7140   -3.3300    0.1450   -0.1210         0         0         0    0.1040;...
  360.0000    2.1520   -5.0000    0.2430   -0.1640         0         0         0    0.0860];
%%%%%%%%%%%%%%%%%%%%%%%%%%%;...

% %%%%%in the x3 direction-sway force coefficients%%%%%%%

%angle(DEGREE)    B0 B1 B2 B3 B4 B5 B6 STANDARD ERROR
B=...
   [0         0         0         0         0         0         0         0         0;...
   10.0000    0.0960    0.2200         0         0         0         0         0    0.0150;...
   20.0000    0.1760    0.7100         0         0         0         0         0    0.0230;...
   30.0000    0.2250    1.3800         0    0.0230         0   -0.2900         0    0.0300;...
   40.0000    0.3290    1.8200         0    0.0430         0   -0.5900         0    0.0540;...
   50.0000    1.1640    1.2600    0.1210         0   -0.2420   -0.9500         0    0.0550;...
   60.0000    1.1630    0.9600    0.1010         0   -0.1770   -0.8800         0    0.0490;...
   70.0000    0.9160    0.5300    0.0690         0         0   -0.6500         0    0.0470;...
   80.0000    0.8440    0.5500    0.0820         0         0   -0.5400         0    0.0460;...
   90.0000    0.8890         0    0.1380         0         0   -0.6600         0    0.0510;...
  100.0000    0.7990         0    0.1550         0         0   -0.5500         0    0.0500;...
  110.0000    0.7970         0    0.1510         0         0   -0.5500         0    0.0490;...
  120.0000    0.9960         0    0.1840         0   -0.2120   -0.6600    0.3400    0.0470;...
  130.0000    1.0140         0    0.1910         0   -0.2800   -0.6900    0.4400    0.0510;...
  140.0000    0.7840         0    0.1660         0   -0.2090   -0.5300    0.3800    0.0600;...
  150.0000    0.5360         0    0.1760   -0.0290   -0.1630         0    0.2700    0.0550;...
  160.0000    0.2510         0    0.1060   -0.0220         0         0         0    0.0360;...
  170.0000    0.1250         0    0.0460   -0.0120         0         0         0    0.0220;...
  180.0000         0         0         0         0         0         0         0         0;...
  190.0000   -0.1250         0   -0.0460    0.0120         0         0         0   -0.0220;...
  200.0000   -0.2510         0   -0.1060    0.0220         0         0         0   -0.0360;...
  210.0000   -0.5360         0   -0.1760    0.0290    0.1630         0   -0.2700   -0.0550;...
  220.0000   -0.7840         0   -0.1660         0    0.2090    0.5300   -0.3800   -0.0600;...
  230.0000   -1.0140         0   -0.1910         0    0.2800    0.6900   -0.4400   -0.0510;...
  240.0000   -0.9960         0   -0.1840         0    0.2120    0.6600   -0.3400   -0.0470;...
  250.0000   -0.7970         0   -0.1510         0         0    0.5500         0   -0.0490;...
  260.0000   -0.7990         0   -0.1550         0         0    0.5500         0   -0.0500;...
  270.0000   -0.8890         0   -0.1380         0         0    0.6600         0   -0.0510;...
  280.0000   -0.8440   -0.5500   -0.0820         0         0    0.5400         0   -0.0460;...
  290.0000   -0.9160   -0.5300   -0.0690         0         0    0.6500         0   -0.0470;...
  300.0000   -1.1630   -0.9600   -0.1010         0    0.1770    0.8800         0   -0.0490;...
  310.0000   -1.1640   -1.2600   -0.1210         0    0.2420    0.9500         0   -0.0550;...
  320.0000   -0.3290   -1.8200         0   -0.0430         0    0.5900         0   -0.0540;...
  330.0000   -0.2250   -1.3800         0   -0.0230         0    0.2900         0   -0.0300;...
  340.0000   -0.1760   -0.7100         0         0         0         0         0   -0.0230;...
  350.0000   -0.0960   -0.2200         0         0         0         0         0   -0.0150;...
  360.0000         0         0         0         0         0         0         0         0];

%%%%%%%%%%%%%%%%%%%%%%%%%%%


% %%%%%in the x2 direction-yaw moment coefficients%%%%%%%

%angle(DEGREE)    C0 C1 C2 C3 C4 C5  STANDARD ERROR
C=...
   [ 0         0         0         0         0         0         0         0;...
   10.0000    0.0596    0.0610         0         0         0   -0.0740    0.0048;...
   20.0000    0.1106    0.2040         0         0         0   -0.1700    0.0074;...
   30.0000    0.2258    0.2450         0         0         0   -0.3800    0.0105;...
   40.0000    0.2017    0.4570         0    0.0067         0   -0.4720    0.0137;...
   50.0000    0.1759    0.5730         0    0.0118         0   -0.5230    0.0149;...
   60.0000    0.1925    0.4800         0    0.0115         0   -0.5460    0.0133;...
   70.0000    0.2133    0.3150         0    0.0081         0   -0.5260    0.0125;...
   80.0000    0.1827    0.2540         0    0.0053         0   -0.4430    0.0123;...
   90.0000    0.2627         0         0         0         0   -0.5080    0.0141;...
  100.0000    0.2102         0   -0.0195         0    0.0335   -0.4920    0.0146;...
  110.0000    0.1567         0   -0.0258         0    0.0497   -0.4570    0.0163;...
  120.0000    0.0801         0   -0.0311         0    0.0740   -0.3960    0.0179;...
  130.0000   -0.0189         0   -0.0488    0.0101    0.1128   -0.4200    0.0166;...
  140.0000    0.0256         0   -0.0422    0.0100    0.0889   -0.4630    0.0162;...
  150.0000    0.0552         0   -0.0381    0.0109    0.0689   -0.4760    0.0141;...
  160.0000    0.0881         0   -0.0306    0.0091    0.0366   -0.4150    0.0105;...
  170.0000    0.0851         0   -0.0122    0.0025         0   -0.2200    0.0057;...
  180.0000         0         0         0         0         0         0         0;...
  190.0000   -0.0851         0    0.0122   -0.0025         0    0.2200   -0.0057;...
  200.0000   -0.0881         0    0.0306   -0.0091   -0.0366    0.4150   -0.0105;...
  210.0000   -0.0552         0    0.0381   -0.0109   -0.0689    0.4760   -0.0141;...
  220.0000   -0.0256         0    0.0422   -0.0100   -0.0889    0.4630   -0.0162;...
  230.0000    0.0189         0    0.0488   -0.0101   -0.1128    0.4200   -0.0166;...
  240.0000   -0.0801         0    0.0311         0   -0.0740    0.3960   -0.0179;...
  250.0000   -0.1567         0    0.0258         0   -0.0497    0.4570   -0.0163;...
  260.0000   -0.2102         0    0.0195         0   -0.0335    0.4920   -0.0146;...
  270.0000   -0.2627         0         0         0         0    0.5080   -0.0141;...
  280.0000   -0.1827   -0.2540         0   -0.0053         0    0.4430   -0.0123;...
  290.0000   -0.2133   -0.3150         0   -0.0081         0    0.5260   -0.0125;...
  300.0000   -0.1925   -0.4800         0   -0.0115         0    0.5460   -0.0133;...
  310.0000   -0.1759   -0.5730         0   -0.0118         0    0.5230   -0.0149;...
  320.0000   -0.2017   -0.4570         0   -0.0067         0    0.4720   -0.0137;...
  330.0000   -0.2258   -0.2450         0         0         0    0.3800   -0.0105;...
  340.0000   -0.1106   -0.2040         0         0         0    0.1700   -0.0074;...
  350.0000   -0.0596   -0.0610         0         0         0    0.0740   -0.0048;...
  360.0000         0         0         0         0         0         0         0];
%%%%%%%%%%%%%%%%%%%%%%%%%%%
Angle=A(:,1);
A0=A(:,2);
A1=A(:,3);
A2=A(:,4);
A3=A(:,5);
A4=A(:,6);
A5=A(:,7);
A6=A(:,8);
A7=A(:,9);

B0=B(:,2);
B1=B(:,3);
B2=B(:,4);
B3=B(:,5);
B4=B(:,6);
B5=B(:,7);
B6=B(:,8);
B7=B(:,9);

C0=C(:,2);
C1=C(:,3);
C2=C(:,4);
C3=C(:,5);
C4=C(:,6);
C5=C(:,7);
C6=C(:,8);

a0 = interp1(Angle,A0,Wind_angle);
a1 = interp1(Angle,A1,Wind_angle);
a2 = interp1(Angle,A2,Wind_angle);
a3 = interp1(Angle,A3,Wind_angle);
a4 = interp1(Angle,A4,Wind_angle);
a5 = interp1(Angle,A5,Wind_angle);
a6 = interp1(Angle,A6,Wind_angle);
a7 = interp1(Angle,A7,Wind_angle);

b0 = interp1(Angle,B0,Wind_angle);
b1 = interp1(Angle,B1,Wind_angle);
b2 = interp1(Angle,B2,Wind_angle);
b3 = interp1(Angle,B3,Wind_angle);
b4 = interp1(Angle,B4,Wind_angle);
b5 = interp1(Angle,B5,Wind_angle);
b6 = interp1(Angle,B6,Wind_angle);
b7 = interp1(Angle,B7,Wind_angle);

c0 = interp1(Angle,C0,Wind_angle);
c1 = interp1(Angle,C1,Wind_angle);
c2 = interp1(Angle,C2,Wind_angle);
c3 = interp1(Angle,C3,Wind_angle);
c4 = interp1(Angle,C4,Wind_angle);
c5 = interp1(Angle,C5,Wind_angle);
c6 = interp1(Angle,C6,Wind_angle);

Cxw=a0+a1*D1+a2*D2+a3*D3+a4*D4+a5*D5+a6*M;
Cyw=b0+b1*D1+b2*D2+b3*D3+b4*D4+b5*D5+b6*D6;
CNw=-(c0+c1*D1+c2*D2+c3*D3+c4*D4+c5*D5);
